simulink subsystem "s2EM"  (R2025b)
settings: Solver=VariableStepAuto  StartTime=0.0  StopTime=10.0  RelTol=1e-3
undefined symbols (not defined in the file): EnvAirTemp, PlntEMCp, PlntEMMass
libraries: autolibutils x1, autolibsharedcommon x1
settings Model: ModifiedByFormat=The MathWorks, Inc.  Creator=The MathWorks, Inc.  LastModifiedBy=The MathWorks, Inc.
settings RTWCC: GPUComputeCapability=3.5

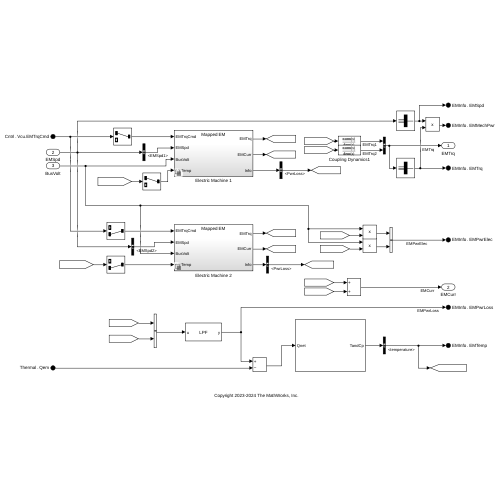
[thumbnail: Simulink's stored preview of the top-level diagram]
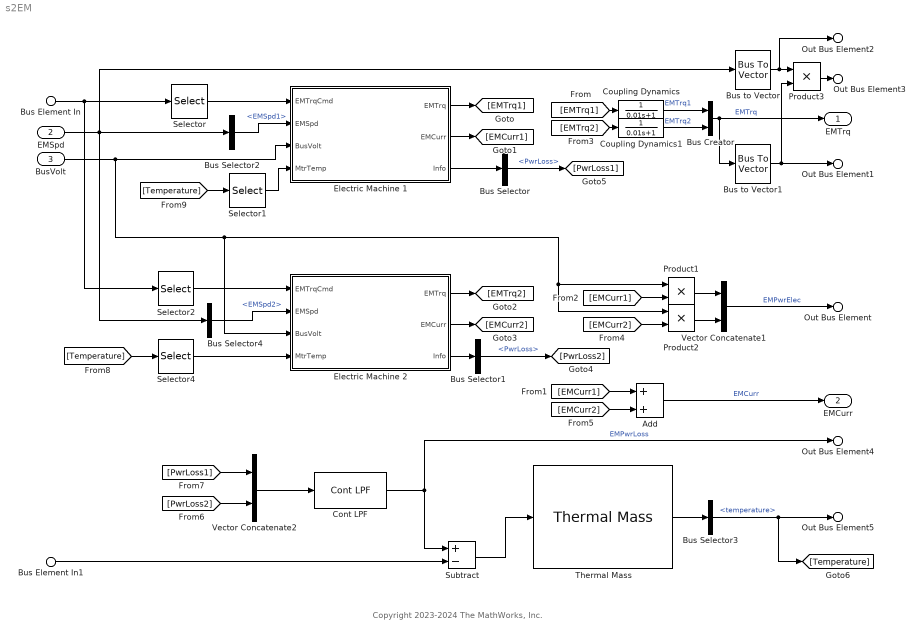
== system s2EM ==
  note: Copyright 2023-2024 The MathWorks, Inc.
  Bus Element In : Inport  PortName=Cntrl  Element=Vcu.EMTrqCmd
  EMSpd : Inport  Port=2
  BusVolt : Inport  Port=3
  Bus Element In1 : Inport  Port=4  PortName=Thermal  Element=Qem
  Add : Sum
  Bus Creator : BusCreator  Inputs=2
  Bus Selector : BusSelector  OutputSignals=PwrLoss
  Bus Selector1 : BusSelector  OutputSignals=PwrLoss
  Bus Selector2 : BusSelector  OutputSignals=EMSpd1
  Bus Selector3 : BusSelector  OutputSignals=temperature
  Bus Selector4 : BusSelector  OutputSignals=EMSpd2
  Bus to Vector : BusToVector
  Bus to Vector1 : BusToVector
  Cont LPF : autolibutils/Cont LPF  wc=1  AbsoluteTolerance=auto  aMode=6
  Coupling Dynamics : TransferFcn  Denominator=[0.01 1]
  Coupling Dynamics1 : TransferFcn  Denominator=[0.01 1]
  Electric Machine 1 : Subsystem  Variant=on  VariantControlMode=label  LabelModeActiveChoice=Mapped EM
  Electric Machine 2 : Subsystem  Variant=on  VariantControlMode=label  LabelModeActiveChoice=Mapped EM
  Product1 : Product
  Product2 : Product
  Product3 : Product
  Selector : Selector  InputPortWidth=2  IndexOptions=Index vector (dialog)  Indices=[1]  OutputSizes=1
  Selector1 : Selector  InputPortWidth=2  IndexOptions=Index vector (dialog)  Indices=[1]  OutputSizes=1
  Selector2 : Selector  InputPortWidth=2  IndexOptions=Index vector (dialog)  Indices=[2]  OutputSizes=1
  Selector4 : Selector  InputPortWidth=2  IndexOptions=Index vector (dialog)  Indices=[2]  OutputSizes=1
  Subtract : Sum  Inputs=+-
  Thermal Mass : autolibsharedcommon/Thermal Mass  MassOrVol=Mass  Mass=PlntEMMass*ones(1,2)  Volume=10  Rho=997  HeatCp=PlntEMCp*ones(1,2)  HeatBrkPts=PlntBattCpBpt  Tinit=EnvAirTemp*ones(1,2)  aMode=6
  Vector Concatenate1 : Concatenate
  Vector Concatenate2 : Concatenate
  EMTrq : Outport
  EMCurr : Outport  Port=2
  Out Bus Element : Outport  Port=3  PortName=EMInfo  Element=EMPwrElec
  Out Bus Element1 : Outport  Port=3  PortName=EMInfo  Element=EMTrq
  Out Bus Element2 : Outport  Port=3  PortName=EMInfo  Element=EMSpd
  Out Bus Element3 : Outport  Port=3  PortName=EMInfo  Element=EMMechPwr
  Out Bus Element4 : Outport  Port=3  PortName=EMInfo  Element=EMPwrLoss
  Out Bus Element5 : Outport  Port=3  PortName=EMInfo  Element=EMTemp
  wires:
  Electric Machine 2/2(EMCurr) -> [EMCurr2]
  Electric Machine 2/1(EMTrq) -> [EMTrq2]
  [EMCurr2] -> Add/2
  [EMCurr2] -> Product2/2
  [EMTrq2] -> Coupling Dynamics1/1
  [EMCurr1] -> Product1/2
  [EMCurr1] -> Add/1
  Electric Machine 1/2(EMCurr) -> [EMCurr1]
  [EMTrq1] -> Coupling Dynamics/1
  Electric Machine 1/1(EMTrq) -> [EMTrq1]
  Selector/1 -> Electric Machine 1/1(EMTrqCmd)
  Add/1 -> EMCurr/1  "EMCurr"
  Selector2/1 -> Electric Machine 2/1(EMTrqCmd)
  Coupling Dynamics1/1 -> Bus Creator/2  "EMTrq2"
  Product2/1 -> Vector Concatenate1/2
  Product1/1 -> Vector Concatenate1/1
  Bus Element In/1 -> Selector/1, Selector2/1
  Vector Concatenate1/1 -> Out Bus Element/1  "EMPwrElec"
  Coupling Dynamics/1 -> Bus Creator/1  "EMTrq1"
  BusVolt/1 -> Electric Machine 1/3(BusVolt), Electric Machine 2/3(BusVolt), Product2/1, Product1/1
  Bus Creator/1 -> Bus to Vector1/1, EMTrq/1  "EMTrq"
  Electric Machine 1/3(Info) -> Bus Selector/1
  Electric Machine 2/3(Info) -> Bus Selector1/1
  Bus Selector1/1 -> [PwrLoss2]  "<PwrLoss>"
  Bus Selector/1 -> [PwrLoss1]  "<PwrLoss>"
  [PwrLoss2] -> Vector Concatenate2/2
  [PwrLoss1] -> Vector Concatenate2/1
  Cont LPF/1 -> Out Bus Element4/1, Subtract/1  "EMPwrLoss"
  Vector Concatenate2/1 -> Cont LPF/1
  Thermal Mass/1 -> Bus Selector3/1
  Bus Selector3/1 -> [Temperature], Out Bus Element5/1  "<temperature>"
  EMSpd/1 -> Bus Selector2/1, Bus Selector4/1, Bus to Vector/1
  Product3/1 -> Out Bus Element3/1
  Bus to Vector/1 -> Out Bus Element2/1, Product3/1
  Bus to Vector1/1 -> Out Bus Element1/1, Product3/2
  Bus Selector2/1 -> Electric Machine 1/2(EMSpd)  "<EMSpd1>"
  Bus Selector4/1 -> Electric Machine 2/2(EMSpd)  "<EMSpd2>"
  Selector1/1 -> Electric Machine 1/4(MtrTemp)
  Selector4/1 -> Electric Machine 2/4(MtrTemp)
  Subtract/1 -> Thermal Mass/1
  Bus Element In1/1 -> Subtract/2
  [Temperature] -> Selector4/1
  [Temperature] -> Selector1/1

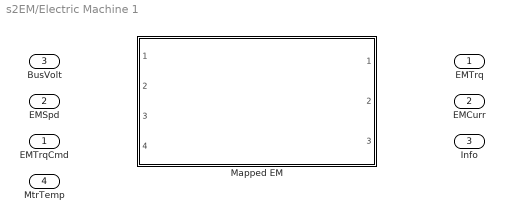
== system s2EM/Electric Machine 1 ==
  EMTrqCmd : Inport
  EMSpd : Inport  Port=2
  BusVolt : Inport  Port=3
  MtrTemp : Inport  Port=4
  Mapped EM : Subsystem  VariantControl=Mapped EM  ReferencedSubsystem=ElectricMachine1
  EMTrq : Outport  VectorParamsAs1DForOutWhenUnconnected=off
  EMCurr : Outport  Port=2  VectorParamsAs1DForOutWhenUnconnected=off
  Info : Outport  Port=3

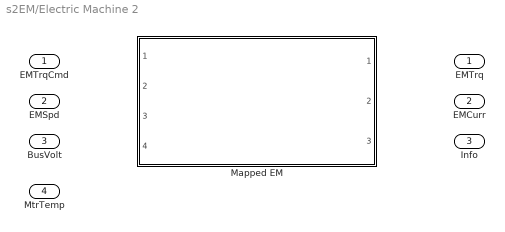
== system s2EM/Electric Machine 2 ==
  EMTrqCmd : Inport
  EMSpd : Inport  Port=2
  BusVolt : Inport  Port=3
  MtrTemp : Inport  Port=4
  Mapped EM : Subsystem  VariantControl=Mapped EM  ReferencedSubsystem=ElectricMachine2
  EMTrq : Outport  VectorParamsAs1DForOutWhenUnconnected=off
  EMCurr : Outport  Port=2  VectorParamsAs1DForOutWhenUnconnected=off
  Info : Outport  Port=3
